simulink library "dspwvfmcdlib"  (Simulink 8.3)
settings: Solver=ode45  SolverMode=SingleTasking  StartTime=0.0  StopTime=10.0  RelTol=1e-3
undefined symbols (not defined in the file): EncIntTau, EncStepAttn, EncStepGain, EncStepInit, EncStepMax, EncStepMin
libraries: dspsigops x8, dspwvfmcdlib x3, dspsigattribs x1
settings Model: RequirementInfo=9  FPTRunName=Active  Creator=The MathWorks Inc.  ExtModeAutoUpdateStatusClock=off

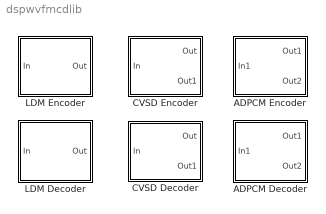
== system dspwvfmcdlib ==
  ADPCM Decoder : Subsystem  mask(ADPCM Decoder){StepAttn=EncStepAttn, StepGain=EncStepGain, StepMax=EncStepMax, StepMin=EncStepMin, StepInit=EncStepInit, AdpcmIntTau=EncIntTau}
      mask prompts: StepAttn "Step-size attenuation"; StepGain "Step-size gain"; StepMax "Maximum step size"; StepMin "Minimum step size"; StepInit "Initial step size"; AdpcmIntTau "Integrator time constant"
      mask Display: disp('ADPCM\nDecoder')
  ADPCM Encoder : Subsystem  mask(ADPCM Encoder){EncStepAttn=.5, EncStepGain=2, EncStepMax=0.5, EncStepMin=0.01, EncStepInit=0.1, EncIntTau=0.99}
      mask prompts: EncStepAttn "Step-size attenuation"; EncStepGain "Step-size gain"; EncStepMax "Maximum step size"; EncStepMin "Minimum step size"; EncStepInit "Initial step size"; EncIntTau "Integrator time constant"
      mask Display: disp('ADPCM\nEncoder')
  CVSD Decoder : Subsystem  mask(CVSD Decoder){DeltaMax=20, SylIntTau=0.99, DeltaMin=0.01, RecIntTau=0.96}
      mask prompts: DeltaMax "Maximum step size"; SylIntTau "Syllabic integrator time constant"; DeltaMin "Minimum step size"; RecIntTau "Reconstruction integrator time constant"
      mask Display: disp('CVSD\nDecoder')
  CVSD Encoder : Subsystem  mask(CVSD Encoder){EncDeltaMax=20, EncSylIntTau=0.99, EncDeltaMin=0.01, EncRecIntTau=0.96}
      mask prompts: EncDeltaMax "Maximum step size"; EncSylIntTau "Syllabic integrator time constant"; EncDeltaMin "Minimum step size"; EncRecIntTau "Reconstruction integrator time constant"
      mask Display: disp('CVSD\nEncoder')
  LDM Decoder : Subsystem  mask(LDM Decoder){Tau=0.91}
      mask prompts: Tau "Integrator time constant"
      mask Display: disp('LDM\nDecoder')
  LDM Encoder : Subsystem  mask(LDM Encoder){EncTau=0.91}
      mask prompts: EncTau "Integrator time constant"
      mask Display: disp('LDM\nEncoder')

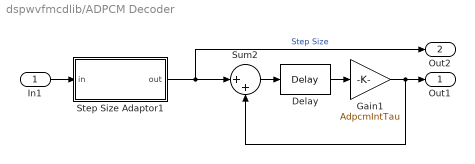
== system dspwvfmcdlib/ADPCM Decoder ==
  In1 : Inport
  Delay : dspsigops/Delay  InputProcessing=Columns as channels (frame based)  dly_unit=Samples  delay=1  ic_detail=on  dif_ic_for_ch=off  dif_ic_for_dly=off  ic=0  reset_popup=None
  Gain1 : Gain  Gain=AdpcmIntTau  SaturateOnIntegerOverflow=on  OutDataTypeStr=Inherit: Same as input  ParamDataTypeStr=Inherit: Same as input
  Step Size Adaptor1 : Subsystem  mask(Step-size adaptation){Dec=StepAttn, Inc=StepGain, MaxStep=StepMax, MinStep=StepMin, InitStep=StepInit}
      mask prompts: Dec "Step-size attenuation factor:"; Inc "Step-size gain factor:"; MaxStep "Maximum step size:"; MinStep "Minimum step size:"; InitStep "Initial step size:"
      mask help: Step-size logic
      mask Display: disp('Step Size\nAdaptation')
  Sum2 : Sum  Inputs=|++  SaturateOnIntegerOverflow=on  InputSameDT=on  OutDataTypeStr=Inherit: Same as first input
  Out1 : Outport
  Out2 : Outport  Port=2
  wires:
  Gain1/1 -> Sum2/2, Out1/1
  Step Size Adaptor1/1(out) -> Out2/1, Sum2/1  "Step Size"
  Sum2/1 -> Delay/1
  Delay/1 -> Gain1/1
  In1/1 -> Step Size Adaptor1/1(in)

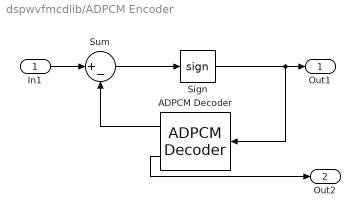
== system dspwvfmcdlib/ADPCM Encoder ==
  In1 : Inport
  ADPCM Decoder : dspwvfmcdlib/ADPCM Decoder  StepAttn=EncStepAttn  StepGain=EncStepGain  StepMax=EncStepMax  StepMin=EncStepMin  StepInit=EncStepInit  AdpcmIntTau=EncIntTau
  Sign : Signum
  Sum : Sum  Inputs=|+-  SaturateOnIntegerOverflow=on  InputSameDT=on  OutDataTypeStr=Inherit: Same as first input
  Out1 : Outport
  Out2 : Outport  Port=2
  wires:
  In1/1 -> Sum/1
  Sign/1 -> Out1/1, ADPCM Decoder/1
  Sum/1 -> Sign/1
  ADPCM Decoder/1 -> Sum/2
  ADPCM Decoder/2 -> Out2/1

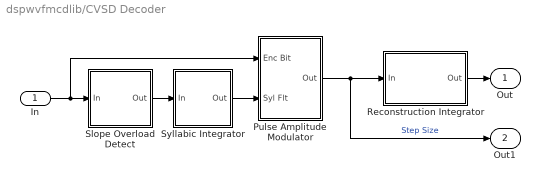
== system dspwvfmcdlib/CVSD Decoder ==
  In : Inport
  Pulse Amplitude Modulator : Subsystem
  Reconstruction Integrator : Subsystem
      mask Display: disp('Reconstruction\nIntegrator')
  Slope Overload Detect : Subsystem
      mask Display: disp('Slope\nOverload\nDetect')
  Syllabic Integrator : Subsystem
      mask Display: disp('Syllabic\nIntegrator')
  Out : Outport
  Out1 : Outport  Port=2
  wires:
  Syllabic Integrator/1(Out) -> Pulse Amplitude Modulator/2(Syl Flt)
  Slope Overload Detect/1(Out) -> Syllabic Integrator/1(In)
  Reconstruction Integrator/1(Out) -> Out/1
  Pulse Amplitude Modulator/1(Out) -> Reconstruction Integrator/1(In), Out1/1  "Step Size"
  In/1 -> Pulse Amplitude Modulator/1(Enc Bit), Slope Overload Detect/1(In)

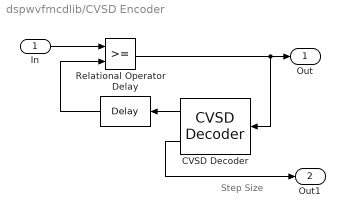
== system dspwvfmcdlib/CVSD Encoder ==
  note: Step Size
  In : Inport
  CVSD Decoder : dspwvfmcdlib/CVSD Decoder  DeltaMax=EncDeltaMax  SylIntTau=EncSylIntTau  DeltaMin=EncDeltaMin  RecIntTau=EncRecIntTau
  Delay : dspsigops/Delay  InputProcessing=Columns as channels (frame based)  dly_unit=Samples  delay=1  ic_detail=on  dif_ic_for_ch=off  dif_ic_for_dly=off  ic=0  reset_popup=None
  Relational Operator : RelationalOperator  InputSameDT=on
  Out : Outport
  Out1 : Outport  Port=2
  wires:
  CVSD Decoder/1 -> Delay/1
  Delay/1 -> Relational Operator/2
  In/1 -> Relational Operator/1
  Relational Operator/1 -> Out/1, CVSD Decoder/1
  CVSD Decoder/2 -> Out1/1

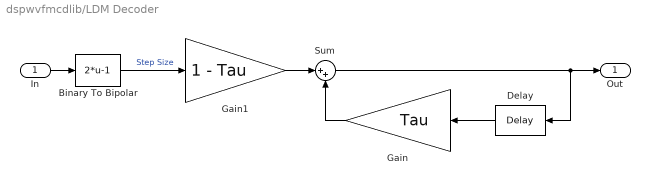
== system dspwvfmcdlib/LDM Decoder ==
  In : Inport
  Binary To Bipolar : Fcn  Expr=2*u-1
  Delay : dspsigops/Delay  InputProcessing=Columns as channels (frame based)  dly_unit=Samples  delay=1  ic_detail=on  dif_ic_for_ch=off  dif_ic_for_dly=off  ic=0  reset_popup=None
  Gain : Gain  Gain=Tau  SaturateOnIntegerOverflow=on  OutDataTypeStr=Inherit: Same as input  ParamDataTypeStr=Inherit: Same as input
  Gain1 : Gain  Gain=1 - Tau  SaturateOnIntegerOverflow=on  OutDataTypeStr=Inherit: Same as input  ParamDataTypeStr=Inherit: Same as input
  Sum : Sum  Inputs=|++  SaturateOnIntegerOverflow=on  InputSameDT=on  OutDataTypeStr=Inherit: Same as first input
  Out : Outport
  wires:
  Binary To Bipolar/1 -> Gain1/1  "Step Size"
  Gain1/1 -> Sum/1
  Sum/1 -> Out/1, Delay/1
  Delay/1 -> Gain/1
  Gain/1 -> Sum/2
  In/1 -> Binary To Bipolar/1

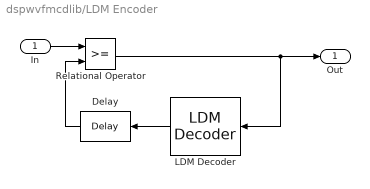
== system dspwvfmcdlib/LDM Encoder ==
  In : Inport
  Delay : dspsigops/Delay  InputProcessing=Columns as channels (frame based)  dly_unit=Samples  delay=1  ic_detail=on  dif_ic_for_ch=off  dif_ic_for_dly=off  ic=0  reset_popup=None
  LDM Decoder : dspwvfmcdlib/LDM Decoder  Tau=EncTau
  Relational Operator : RelationalOperator  InputSameDT=on
  Out : Outport
  wires:
  LDM Decoder/1 -> Delay/1
  Relational Operator/1 -> LDM Decoder/1, Out/1
  Delay/1 -> Relational Operator/2
  In/1 -> Relational Operator/1

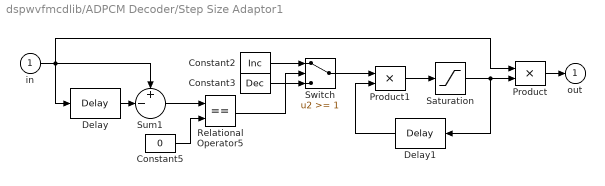
== system dspwvfmcdlib/ADPCM Decoder/Step Size Adaptor1 ==
  in : Inport
  Constant2 : Constant  Value=Inc
  Constant3 : Constant  Value=Dec
  Constant5 : Constant  Value=0
  Delay : dspsigops/Delay  InputProcessing=Columns as channels (frame based)  dly_unit=Samples  delay=1  ic_detail=on  dif_ic_for_ch=off  dif_ic_for_dly=off  ic=0  reset_popup=None
  Delay1 : dspsigops/Delay  InputProcessing=Columns as channels (frame based)  dly_unit=Samples  delay=1  ic_detail=on  dif_ic_for_ch=off  dif_ic_for_dly=off  ic=InitStep  reset_popup=None
  Product : Product  SaturateOnIntegerOverflow=on  RndMeth=Zero  InputSameDT=on  OutDataTypeStr=Inherit: Same as first input
  Product1 : Product  SaturateOnIntegerOverflow=on  RndMeth=Zero  InputSameDT=on  OutDataTypeStr=Inherit: Same as first input
  Relational Operator5 : RelationalOperator  Operator===  InputSameDT=on
  Saturation : Saturate  UpperLimit=MaxStep  LowerLimit=MinStep
  Sum1 : Sum  Inputs=+-|  SaturateOnIntegerOverflow=on  InputSameDT=on  OutDataTypeStr=Inherit: Same as first input
  Switch : Switch  Threshold=1  SaturateOnIntegerOverflow=on  InputSameDT=on
  out : Outport  InitialOutput=0
  wires:
  Saturation/1 -> Product/2, Delay1/1
  Product/1 -> out/1
  Relational Operator5/1 -> Switch/2
  Constant2/1 -> Switch/1
  Constant3/1 -> Switch/3
  Sum1/1 -> Relational Operator5/1
  Product1/1 -> Saturation/1
  Switch/1 -> Product1/1
  Delay1/1 -> Product1/2
  in/1 -> Sum1/1, Product/1, Delay/1
  Delay/1 -> Sum1/2
  Constant5/1 -> Relational Operator5/2

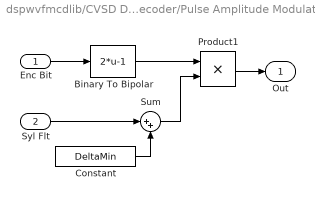
== system dspwvfmcdlib/CVSD Decoder/Pulse Amplitude Modulator ==
  Enc Bit : Inport
  Syl Flt : Inport  Port=2
  Binary To Bipolar : Fcn  Expr=2*u-1
  Constant : Constant  Value=DeltaMin
  Product1 : Product  SaturateOnIntegerOverflow=on  RndMeth=Zero  InputSameDT=on  OutDataTypeStr=Inherit: Same as first input
  Sum : Sum  Inputs=|++  SaturateOnIntegerOverflow=on  InputSameDT=on  OutDataTypeStr=Inherit: Same as first input
  Out : Outport
  wires:
  Enc Bit/1 -> Binary To Bipolar/1
  Binary To Bipolar/1 -> Product1/1
  Sum/1 -> Product1/2
  Syl Flt/1 -> Sum/1
  Constant/1 -> Sum/2
  Product1/1 -> Out/1

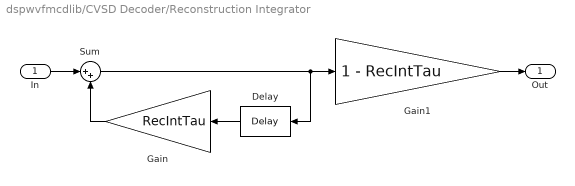
== system dspwvfmcdlib/CVSD Decoder/Reconstruction Integrator ==
  In : Inport
  Delay : dspsigops/Delay  InputProcessing=Columns as channels (frame based)  dly_unit=Samples  delay=1  ic_detail=on  dif_ic_for_ch=off  dif_ic_for_dly=off  ic=0  reset_popup=None
  Gain : Gain  Gain=RecIntTau  SaturateOnIntegerOverflow=on  OutDataTypeStr=Inherit: Same as input  ParamDataTypeStr=Inherit: Same as input
  Gain1 : Gain  Gain=1 - RecIntTau  SaturateOnIntegerOverflow=on  OutDataTypeStr=Inherit: Same as input  ParamDataTypeStr=Inherit: Same as input
  Sum : Sum  Inputs=|++  SaturateOnIntegerOverflow=on  InputSameDT=on  OutDataTypeStr=Inherit: Same as first input
  Out : Outport
  wires:
  Gain1/1 -> Out/1
  Gain/1 -> Sum/2
  Delay/1 -> Gain/1
  Sum/1 -> Gain1/1, Delay/1
  In/1 -> Sum/1

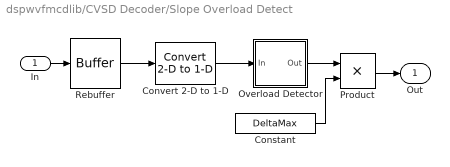
== system dspwvfmcdlib/CVSD Decoder/Slope Overload Detect ==
  In : Inport
  Constant : Constant  Value=DeltaMax
  Convert 2-D to 1-D : dspsigattribs/Convert 2-D to 1-D
  Overload Detector : Subsystem
      mask Display: disp('Overload\nDetector')
  Product : Product  SaturateOnIntegerOverflow=on  RndMeth=Zero  InputSameDT=on  OutDataTypeStr=Inherit: Same as first input
  Rebuffer : Buffer  N=3  V=2  TreatMby1Signals=One channel
  Out : Outport
  wires:
  Rebuffer/1 -> Convert 2-D to 1-D/1
  Overload Detector/1(Out) -> Product/1
  Constant/1 -> Product/2
  In/1 -> Rebuffer/1
  Product/1 -> Out/1
  Convert 2-D to 1-D/1 -> Overload Detector/1(In)

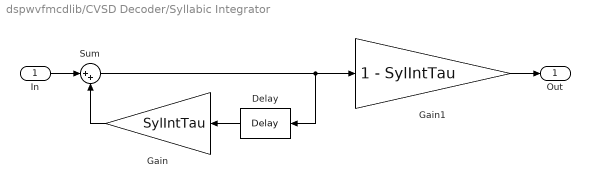
== system dspwvfmcdlib/CVSD Decoder/Syllabic Integrator ==
  In : Inport
  Delay : dspsigops/Delay  InputProcessing=Columns as channels (frame based)  dly_unit=Samples  delay=1  ic_detail=on  dif_ic_for_ch=off  dif_ic_for_dly=off  ic=0  reset_popup=None
  Gain : Gain  Gain=SylIntTau  SaturateOnIntegerOverflow=on  OutDataTypeStr=Inherit: Same as input  ParamDataTypeStr=Inherit: Same as input
  Gain1 : Gain  Gain=1 - SylIntTau  SaturateOnIntegerOverflow=on  OutDataTypeStr=Inherit: Same as input  ParamDataTypeStr=Inherit: Same as input
  Sum : Sum  Inputs=|++  SaturateOnIntegerOverflow=on  InputSameDT=on  OutDataTypeStr=Inherit: Same as first input
  Out : Outport
  wires:
  Gain1/1 -> Out/1
  Gain/1 -> Sum/2
  Delay/1 -> Gain/1
  Sum/1 -> Gain1/1, Delay/1
  In/1 -> Sum/1

== system dspwvfmcdlib/CVSD Decoder/Slope Overload Detect/Overload Detector ==
  In : Inport
  111 Overload Detection : Logic  Inputs=1
  111 Overload Detection1 : Logic  Operator=NOR  Inputs=1
  Slope Overload Detection1 : Logic  Operator=OR
  Out : Outport
  wires:
  Slope Overload Detection1/1 -> Out/1
  In/1 -> 111 Overload Detection1/1, 111 Overload Detection/1
  111 Overload Detection1/1 -> Slope Overload Detection1/2
  111 Overload Detection/1 -> Slope Overload Detection1/1
